simulink model "HybridPowertrain_TestBench_Final"  (R2017a)
settings: Solver=ode1  StartTime=0.0  StopTime=1400  FixedStep=0.01  RelTol=1e-3  EnableMultiTasking=on
undefined symbols (not defined in the file): AccActPos, air, Atm_temp, bms_inletair_temp, BMS_IstStrom, bms_maxchargecurrent, bms_maxdischargecurrent, BMS_Notfallkuehlung, BMS_SOC, BrkPdlPos, cal, Cells, Chg, D1_Commanded_Torque, D1_DC_Bus_Voltage, D2_Motor_Speed, D2_Torque_Feedback, DriverControls, EcoCAR3_Lib, Em, EngActStdyStTorq, Engine, EngSpd, env, ESS, fd, g, gb, Gearbox, GearBox, gps_lat, gps_long, Grade, I_loss, IMG, InstFuelConsmpRate, KeyPosition, lib_ESS_plant_V1_2, Loss, max_vehicle_rad_air_flow, mot, mph2kph, mph2ms, NeutralGear, ParkGear, PPEI_Engine_General_Status_2__ThrPos, PTEI_Engine_Torque_Status__EngActStdyStTorq, R_0, R_1, Ratio, RegenBrkDisable, rho, SampleTime, ShiftLeverPosition, SOC_bp, SOC_init, Spd, Speed, SW_CS_ON, SW_Engine_ON ... (+15)
libraries: simulink x39, fl_lib x13, nesl_utility x8, Utility x1, EC2_libraries x1
(part 3 of 5)

== system HybridPowertrain_TestBench_Final/ESS/Soft BMS/BMS_1 ==
  Bus Creator8 : BusCreator  Inputs=9
  Constant2 : Constant  Value=0
  BMS_06 : Outport
  wires:
  ? -> Bus Creator8/5
  ? -> Bus Creator8/9
  ? -> Bus Creator8/7
  ? -> Bus Creator8/3
  ? -> Bus Creator8/4
  ? -> Bus Creator8/6
  ? -> Bus Creator8/8
  Bus Creator8/1 -> BMS_06/1  "BMS_06"
  Constant2/1 -> Bus Creator8/2  "BMS_SollVolumenStrom"

== system HybridPowertrain_TestBench_Final/ESS/Soft BMS/BMS_2 ==
  Bus Creator8 : BusCreator  Inputs=9
  BMS_07 : Outport
  wires:
  ? -> Bus Creator8/2
  Bus Creator8/1 -> BMS_07/1  "BMS_07"
  ? -> Bus Creator8/8
  ? -> Bus Creator8/6
  ? -> Bus Creator8/4
  ? -> Bus Creator8/3
  [BMS_Gesamtst_Spgfreiheit] -> Bus Creator8/1  "BMS_Gesamtst_Spgfreiheit"
  ? -> Bus Creator8/7
  ? -> Bus Creator8/9
  ? -> Bus Creator8/5

== system HybridPowertrain_TestBench_Final/ESS/Soft BMS/BMS_3 ==
  Bus Creator8 : BusCreator  Inputs=3
  Constant : Constant  Value=255
  Constant1 : Constant  Value=254
  Data Type Conversion : DataTypeConversion
  ISO_Hybrid_01_Resp : Outport
  wires:
  Bus Creator8/1 -> ISO_Hybrid_01_Resp/1  "ISO_Hybrid_01_Resp"
  Data Type Conversion/1 -> Bus Creator8/1  "ISO_Hybrid_01_Resp_Data_4"
  Constant/1 -> Bus Creator8/2  "ISO_Hybrid_01_Resp_Data_5"
  Constant1/1 -> Bus Creator8/3  "ISO_Hybrid_01_Resp_Data_6"
  [ISO_Hybrid_01_Req_Data_4] -> Data Type Conversion/1  "ISO_Hybrid_01_Resp_Data_4"

== system HybridPowertrain_TestBench_Final/ESS/Soft BMS/BMS_HYB_1 ==
  BMS_HYB_02_BZ : Subsystem
  Bus Creator3 : BusCreator  Inputs=20
  Clock3 : Clock  Commented=on
  Constant12 : Constant  Value=0
  Constant7 : Constant  Value=0
  Constant8 : Constant  Value=0
  Data Type Conversion : DataTypeConversion
  Speed1 : Lookup  Commented=on  InputValues=[0 75 75 100 100 120]  Table=[0 0 1 1 0 0]
  BMS_HYB_02 : Outport
  wires:
  [BMS_SleepInd] -> Bus Creator3/17  "BMS_SleepInd"
  [BMS_Fehler_Notabschaltung_Pilot] -> Bus Creator3/16  "BMS_Fehler_Notabschaltung_Pilot"
  [BMS_Init_abgeschlossen] -> Bus Creator3/15  "BMS_Init_abgeschlossen"
  Constant12/1 -> Bus Creator3/14  "BMS_Fehler_Kaltstartleistung"
  [BMS_IstSpannung] -> Bus Creator3/13  "BMS_IstSpannung"
  [BMS_Fehler_verschweisst] -> Bus Creator3/12  "BMS_Fehler_HS_verschweisst"
  [BMS_Fehler_HS_offen] -> Bus Creator3/11  "BMS_Fehler_HS_offen"
  [BMS_IstStrom] -> Bus Creator3/10  "BMS_IstStrom"
  [BMS_Fehler_Pilot] -> Bus Creator3/9  "BMS_Fehler_Pilot"
  [BMS_Gesamtst_Spgfreiheit] -> Bus Creator3/4  "BMS_Status_Spgfreiheit"
  [BMS_Fehler_Notabschaltung_Crash] -> Bus Creator3/5  "BMS_Fehler_Notabschaltung_Crash"
  Constant8/1 -> Bus Creator3/8  "BMS_Fehler_Isolation"
  [BMS_Notfallkuehlung] -> Bus Creator3/2  "BMS_Notfallkuehlung"
  Constant7/1 -> Bus Creator3/7  "BMS_Fehler_HVBattAbschaltung_Anf"
  [BMS_Fehler_Notabschaltung_Crash] -> Bus Creator3/6  "BMS_Fehler_HVBattAbschaltung"
  [BMS_Gesamtst_Spgfreiheit] -> Bus Creator3/3  "BMS_Status_Spannungsfreiheit"
  Data Type Conversion/1 -> Bus Creator3/1  "BMS_IstModus"
  Bus Creator3/1 -> BMS_HYB_02/1  "BMS_HYB_02"
  Clock3/1 -> Speed1/1
  [BMS_IstModus] -> Data Type Conversion/1  "BMS_IstModus"
  BMS_HYB_02_BZ/1(Out1) -> Bus Creator3/18

== system HybridPowertrain_TestBench_Final/ESS/Soft BMS/BMS_HYB_2 ==
  Bus Creator3 : BusCreator  Inputs=10
  Data Type Conversion : DataTypeConversion
  BMS_HYB_03 : Outport
  wires:
  Bus Creator3/1 -> BMS_HYB_03/1  "BMS_HYB_03"
  Data Type Conversion/1 -> Bus Creator3/1  "BMS_SOC"
  [BMS_SOC] -> Data Type Conversion/1  "BMS_SOC"

== system HybridPowertrain_TestBench_Final/ESS/Soft BMS/BMS_HYB_3 ==
  Bus Creator6 : BusCreator  Inputs=9
  Constant : Constant
  Constant1 : Constant  Commented=on  Value=bms_maxdischargecurrent
  Constant2 : Constant
  Constant3 : Constant  Commented=on  Value=bms_maxchargecurrent
  BMS_HYB_04 : Outport
  wires:
  Constant2/1 -> Bus Creator6/2
  [BMS_Spannung_ZwKr] -> Bus Creator6/3  "BMS_Spannung_ZwKr"
  ? -> Bus Creator6/7
  ? -> Bus Creator6/9
  ? -> Bus Creator6/8
  ? -> Bus Creator6/5
  ? -> Bus Creator6/4
  ? -> Bus Creator6/6
  Bus Creator6/1 -> BMS_HYB_04/1  "BMS_HYB_04"
  Constant/1 -> Bus Creator6/1  "BMS_MaxDyn_LadeStrom"

== system HybridPowertrain_TestBench_Final/ESS/Soft BMS/BMS_HYB_4 ==
  Bus Creator6 : BusCreator  Inputs=9
  Constant1 : Constant  Value=430
  Constant2 : Constant  Value=291
  Constant3 : Constant  Value=0
  Constant4 : Constant  Commented=on  Value=bms_inletair_temp
  Constant5 : Constant  Value=20
  BMS_HYB_06 : Outport
  wires:
  Constant5/1 -> Bus Creator6/5  "BMS_Temperatur_Ansaugluft"
  [BMS_Temperatur] -> Bus Creator6/4  "BMS_Temperatur"
  Constant3/1 -> Bus Creator6/1  "BMS_Balancing_Anf"
  Bus Creator6/1 -> BMS_HYB_06/1  "BMS_HYB_06"
  ? -> Bus Creator6/6
  Constant2/1 -> Bus Creator6/3  "BMS_Min_EntladeSpannung"
  ? -> Bus Creator6/8
  ? -> Bus Creator6/9
  ? -> Bus Creator6/7
  Constant1/1 -> Bus Creator6/2  "BMS_Max_LadeSpannung"

== system HybridPowertrain_TestBench_Final/ESS/Soft BMS/BMS_HYB_5 ==
  Bus Creator6 : BusCreator  Inputs=9
  BMS_HYB_07 : Outport
  wires:
  ? -> Bus Creator6/7
  ? -> Bus Creator6/9
  ? -> Bus Creator6/8
  ? -> Bus Creator6/5
  ? -> Bus Creator6/4
  ? -> Bus Creator6/6
  Bus Creator6/1 -> BMS_HYB_07/1  "BMS_HYB_07"
  [BMS_Temperierung_Anf] -> Bus Creator6/1  "BMS_Temperierung_Anf"

== system HybridPowertrain_TestBench_Final/ESS/Soft BMS/BMS_Hybrid_1 ==
  Bus Creator8 : BusCreator  Inputs=1
  BMS_Hybrid_01 : Outport
  wires:
  [BMS_HYB_Kuehlung_Anf] -> Bus Creator8/1  "BMS_HYB_Kuehlung_Anf"
  Bus Creator8/1 -> BMS_Hybrid_01/1  "BMS_Hybrid_01"

== system HybridPowertrain_TestBench_Final/ESS/Soft BMS/Energy Consumption ==
  Current : Inport
  Voltage : Inport  Port=2
  Divide : Product  Inputs=*/
  Divide by zero : Subsystem
  Gain : Gain  Gain=mph2kph
  Initial Current1 : Memory  InheritSampleTime=on
  Multiply : Product  Inputs=**
  Sum5 : Sum  Inputs=|++  SaturateOnIntegerOverflow=on  InputSameDT=on  OutDataTypeStr=Inherit: Same as first input
  To Workspace4 : ToWorkspace  VariableName=ess_wh_per_km  SampleTime=-1
      settings: Decimation=WORKSPACE_DECIMATION
  To_WHr1 : Gain  Gain=tloop/3600  SaturateOnIntegerOverflow=on  OutDataTypeStr=Inherit: Same as input  ParamDataTypeStr=Inherit: Same as input
  tag scope: ESSPwr=global
  wires:
  Current/1 -> Multiply/1
  Voltage/1 -> Multiply/2
  Multiply/1 -> [ESSPwr], To_WHr1/1  "Power"
  To_WHr1/1 -> Sum5/1  "d(Wh)"
  Sum5/1 -> Initial Current1/1  "Wh"
  Initial Current1/1 -> Sum5/2, Divide/1  "Wh"
  [veh_dist_miles] -> Gain/1  "mi"
  Divide/1 -> To Workspace4/1  "Wh/km"
  Gain/1 -> Divide by zero/1(In1)  "km"
  Divide by zero/1(Out1) -> Divide/2

== system HybridPowertrain_TestBench_Final/ESS/Soft BMS/HV_Netz status ==
  ess_vbat : Inport
  Constant3 : Constant  Value=2
  Constant4 : Constant
  Constant5 : Constant  Value=0
  Constant6 : Constant  Value=0
  Memory : Memory
  Memory1 : Memory
  Switch : Switch  Criteria=u2 > Threshold  Threshold=20
  Switch1 : Switch  Threshold=1
  Switch2 : Switch  Threshold=7
  BMS_Spannung_Zwkr : Outport
  BMS_Gesamtst_Spgfreiheit : Outport  Port=2
  wires:
  Constant5/1 -> Switch1/3
  [BMS_IstModus] -> Switch1/2, Switch2/2
  Switch1/1 -> Memory/1
  Constant6/1 -> Switch2/1
  Switch2/1 -> Memory1/1
  Constant4/1 -> Switch/3
  Switch/1 -> BMS_Gesamtst_Spgfreiheit/1
  Constant3/1 -> Switch/1
  ess_vbat/1 -> Switch1/1
  Memory/1 -> Switch2/3
  Memory1/1 -> BMS_Spannung_Zwkr/1, Switch/2

== system HybridPowertrain_TestBench_Final/ESS/Soft BMS/Limits ==
  vcell : Inport
  Average Current : Subsystem
  Compare To Constant1 : simulink/Logic and Bit Operations/Compare To Constant  relop=<=  const=3.0  OutDataTypeStr=boolean
  Compare To Constant2 : simulink/Logic and Bit Operations/Compare To Constant  relop=<=  const=3.0  OutDataTypeStr=boolean
  Constant3 : Constant  Value=25
  Derate : Subsystem
  Derate2 : Subsystem
  Gain : Gain  Gain=1/1.9
  Gain1 : Gain  Gain=1/1.9
  To Workspace10 : ToWorkspace  VariableName=ess_dis_max_current_underated  SampleTime=-1
      settings: Decimation=WORKSPACE_DECIMATION
  To Workspace3 : ToWorkspace  VariableName=ess_dis_max  SampleTime=-1
      settings: Decimation=WORKSPACE_DECIMATION
  To Workspace4 : ToWorkspace  VariableName=ess_chg_max  SampleTime=-1
      settings: Decimation=WORKSPACE_DECIMATION
  To Workspace9 : ToWorkspace  VariableName=ess_chg_max_current_underated  SampleTime=-1
      settings: Decimation=WORKSPACE_DECIMATION
  bcm_chg_max_tbl : Lookup2D  RowIndex=ess.plant.init.limit.idx1_soc  ColumnIndex=ess.plant.init.limit.idx2_temp  Table=ess.plant.init.max_charge_limit
  bcm_dis_max_tbl : Lookup2D  RowIndex=ess.plant.init.limit.idx1_soc  ColumnIndex=ess.plant.init.limit.idx2_temp  Table=ess.plant.init.max_discharge_limit
  bcm_dis_max : Outport
  bcm_chg_max : Outport  Port=2
  Discharge Buffer : Outport  Port=3
  Charge Buffer : Outport  Port=4
  t_coolant : Outport  Port=5
  undervolt : Outport  Port=6
  overvolt : Outport  Port=7
  tag scope: bcm_chg_max=global
  wires:
  [BMS_Temperatur] -> bcm_chg_max_tbl/2, bcm_dis_max_tbl/2, Average Current/2(Temp)
  bcm_dis_max_tbl/1 -> Gain/1
  Derate/1(Derate) -> bcm_dis_max/1, To Workspace3/1
  bcm_chg_max_tbl/1 -> Gain1/1  "bcm_chg_max"
  Derate2/1(Derate) -> To Workspace4/1, [bcm_chg_max], bcm_chg_max/1
  [BMS_SOC] -> Average Current/1(SOC), bcm_dis_max_tbl/1, bcm_chg_max_tbl/1
  Average Current/1(Discharge Buffer) -> Derate/2(Buffer), Discharge Buffer/1
  Average Current/2(Discharge Cont) -> Derate/3(Cont Current)
  Average Current/3(Charge Buffer) -> Derate2/1(Buffer), Charge Buffer/1
  Average Current/4(Charge Cont) -> Derate2/2(Cont Current)
  vcell/1 -> Compare To Constant1/1, Compare To Constant2/1
  Constant3/1 -> t_coolant/1
  Compare To Constant2/1 -> overvolt/1
  Compare To Constant1/1 -> undervolt/1
  Gain/1 -> Derate/1(Current Limit), To Workspace10/1
  Gain1/1 -> To Workspace9/1, Derate2/3(Current Limit)

== system HybridPowertrain_TestBench_Final/ESS/Soft BMS/NMH_BMS1 ==
  Bus Creator8 : BusCreator  Inputs=9
  NMH_BMS : Outport
  wires:
  [NMH_BMS_Start_1] -> Bus Creator8/3  "NMH_BMS_Start_1"
  [NMH_BMS_Normal_Mode_2] -> Bus Creator8/2  "NMH_BMS_Normal_Mode_2"
  Bus Creator8/1 -> NMH_BMS/1  "NMH_BMS"
  ? -> Bus Creator8/8
  ? -> Bus Creator8/6
  [NMH_BMS_Start_2] -> Bus Creator8/4  "NMH_BMS_Start_2"
  [NMH_BMS_Normal_Mode_1] -> Bus Creator8/1  "NMH_BMS_Normal_Mode_1"
  ? -> Bus Creator8/7
  ? -> Bus Creator8/9
  [NMH_BMS_Car_WakeUp] -> Bus Creator8/5  "NMH_BMS_Car_WakeUp"

== system HybridPowertrain_TestBench_Final/ESS/Soft BMS/NoiseAdd ==
  In : Inport
  Random Number : RandomNumber  Variance=0.1  SampleTime=tloop
  Rate Transition : RateTransition
  Sum : Sum  Inputs=|++
  Out : Outport
  wires:
  Random Number/1 -> Rate Transition/1
  In/1 -> Sum/1
  Sum/1 -> Out/1
  Rate Transition/1 -> Sum/2

== system HybridPowertrain_TestBench_Final/ESS/Soft BMS/RollingAliveCnt1 ==
  Constant : Constant
  Rolling Alive Counter : Stateflow chart  TreatAsAtomicUnit=on
  Switch : Switch  Criteria=u2 > Threshold
  Out1 : Outport
  wires:
  Switch/1 -> Out1/1
  [BMS_CAN_fault] -> Switch/2
  Rolling Alive Counter/1(RollingAliveCnt) -> Switch/3
  Constant/1 -> Switch/1

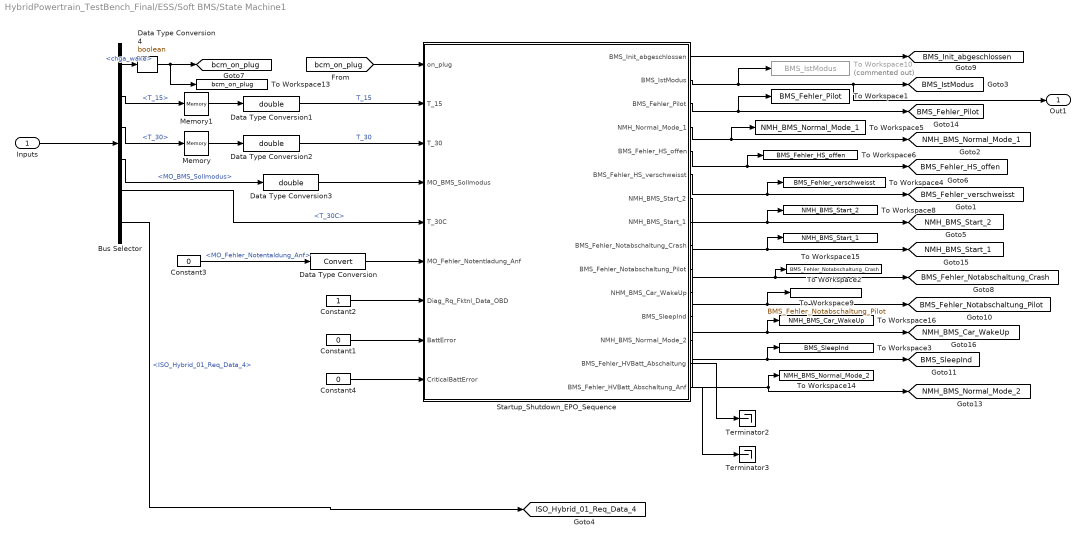
== system HybridPowertrain_TestBench_Final/ESS/Soft BMS/State Machine1 ==
  Inputs : Inport
  Bus Selector : BusSelector  OutputSignals=chga_wake,T_15,T_30,MO_BMS_Sollmodus,T_30C,ISO_Hybrid_01_Req_Data_4
  Constant1 : Constant  Value=0  OutDataTypeStr=boolean
  Constant2 : Constant  OutDataTypeStr=boolean
  Constant3 : Constant  Value=0  OutDataTypeStr=boolean
  Constant4 : Constant  Value=0  OutDataTypeStr=boolean
  Data Type Conversion : DataTypeConversion
  Data Type Conversion1 : DataTypeConversion  OutDataTypeStr=double
  Data Type Conversion2 : DataTypeConversion  OutDataTypeStr=double
  Data Type Conversion3 : DataTypeConversion  OutDataTypeStr=double
  Data Type Conversion4 : DataTypeConversion  OutDataTypeStr=boolean
  Memory : Memory  InheritSampleTime=on
  Memory1 : Memory  InheritSampleTime=on
  Startup_Shutdown_EPO_Sequence : Stateflow chart  TreatAsAtomicUnit=on
  Terminator2 : Terminator
  Terminator3 : Terminator
  To Workspace1 : ToWorkspace  VariableName=BMS_Fehler_Pilot  SampleTime=-1
      settings: Decimation=WORKSPACE_DECIMATION
  To Workspace10 : ToWorkspace  Commented=on  VariableName=BMS_IstModus  SampleTime=-1
      settings: Decimation=WORKSPACE_DECIMATION
  To Workspace13 : ToWorkspace  VariableName=bcm_on_plug  SampleTime=-1
      settings: Decimation=WORKSPACE_DECIMATION
  To Workspace14 : ToWorkspace  VariableName=NMH_BMS_Normal_Mode_2  SampleTime=-1
      settings: Decimation=WORKSPACE_DECIMATION
  To Workspace15 : ToWorkspace  VariableName=NMH_BMS_Start_1  SampleTime=-1
      settings: Decimation=WORKSPACE_DECIMATION
  To Workspace16 : ToWorkspace  VariableName=NMH_BMS_Car_WakeUp  SampleTime=-1
      settings: Decimation=WORKSPACE_DECIMATION
  To Workspace2 : ToWorkspace  VariableName=BMS_Fehler_Notabschaltung_Crash  SampleTime=-1
      settings: Decimation=WORKSPACE_DECIMATION
  To Workspace3 : ToWorkspace  VariableName=BMS_SleepInd  SampleTime=-1
      settings: Decimation=WORKSPACE_DECIMATION
  To Workspace4 : ToWorkspace  VariableName=BMS_Fehler_verschweisst  SampleTime=-1
      settings: Decimation=WORKSPACE_DECIMATION
  To Workspace5 : ToWorkspace  VariableName=NMH_BMS_Normal_Mode_1  SampleTime=-1
      settings: Decimation=WORKSPACE_DECIMATION
  To Workspace6 : ToWorkspace  VariableName=BMS_Fehler_HS_offen  SampleTime=-1
      settings: Decimation=WORKSPACE_DECIMATION
  To Workspace8 : ToWorkspace  VariableName=NMH_BMS_Start_2  SampleTime=-1
      settings: Decimation=WORKSPACE_DECIMATION
  To Workspace9 : ToWorkspace  VariableName=BMS_Fehler_Notabschaltung_Pilot  SampleTime=-1
      settings: Decimation=WORKSPACE_DECIMATION
  Out1 : Outport
  tag scope: BMS_Fehler_HS_offen=global, BMS_Fehler_Notabschaltung_Crash=global, BMS_Fehler_Notabschaltung_Pilot=global, BMS_Fehler_Pilot=global, BMS_Fehler_verschweisst=global, BMS_Init_abgeschlossen=global, BMS_IstModus=global, BMS_SleepInd=global, ISO_Hybrid_01_Req_Data_4=global, NMH_BMS_Car_WakeUp=global, NMH_BMS_Normal_Mode_1=global, NMH_BMS_Normal_Mode_2=global, NMH_BMS_Start_1=global, NMH_BMS_Start_2=global, bcm_on_plug=global
  wires:
  Data Type Conversion4/1 -> [bcm_on_plug], To Workspace13/1
  Data Type Conversion3/1 -> Startup_Shutdown_EPO_Sequence/4(MO_BMS_Sollmodus)
  Memory1/1 -> Data Type Conversion1/1
  Memory/1 -> Data Type Conversion2/1
  Data Type Conversion2/1 -> Startup_Shutdown_EPO_Sequence/3(T_30)  "T_30"
  Data Type Conversion1/1 -> Startup_Shutdown_EPO_Sequence/2(T_15)  "T_15"
  Data Type Conversion/1 -> Startup_Shutdown_EPO_Sequence/6(MO_Fehler_Notentladung_Anf)
  Bus Selector/4 -> Data Type Conversion3/1  "<MO_BMS_Sollmodus>"
  Inputs/1 -> Bus Selector/1
  Startup_Shutdown_EPO_Sequence/15(BMS_Fehler_HVBatt_Abschaltung_Anf) -> Terminator3/1
  Startup_Shutdown_EPO_Sequence/14(BMS_Fehler_HVBatt_Abschaltung) -> Terminator2/1
  Constant4/1 -> Startup_Shutdown_EPO_Sequence/9(CriticalBattError)
  Constant2/1 -> Startup_Shutdown_EPO_Sequence/7(Diag_Rq_Fktnl_Data_OBD)
  Constant1/1 -> Startup_Shutdown_EPO_Sequence/8(BattError)
  Constant3/1 -> Data Type Conversion/1  "<MO_Fehler_Notentaldung_Anf>"
  Bus Selector/5 -> Startup_Shutdown_EPO_Sequence/5(T_30C)  "<T_30C>"
  [bcm_on_plug] -> Startup_Shutdown_EPO_Sequence/1(on_plug)
  Startup_Shutdown_EPO_Sequence/11(NHM_BMS_Car_WakeUp) -> [NMH_BMS_Car_WakeUp], To Workspace16/1
  Startup_Shutdown_EPO_Sequence/8(NMH_BMS_Start_1) -> To Workspace15/1, [NMH_BMS_Start_1]
  Startup_Shutdown_EPO_Sequence/7(NMH_BMS_Start_2) -> [NMH_BMS_Start_2], To Workspace8/1
  Startup_Shutdown_EPO_Sequence/13(NMH_BMS_Normal_Mode_2) -> [NMH_BMS_Normal_Mode_2], To Workspace14/1
  Startup_Shutdown_EPO_Sequence/3(BMS_Fehler_Pilot) -> [BMS_Fehler_Pilot], To Workspace1/1
  Startup_Shutdown_EPO_Sequence/1(BMS_Init_abgeschlossen) -> [BMS_Init_abgeschlossen]
  Startup_Shutdown_EPO_Sequence/2(BMS_IstModus) -> To Workspace10/1, [BMS_IstModus], Out1/1
  Bus Selector/2 -> Memory1/1  "<T_15>"
  Startup_Shutdown_EPO_Sequence/6(BMS_Fehler_HS_verschweisst) -> To Workspace4/1, [BMS_Fehler_verschweisst]
  Startup_Shutdown_EPO_Sequence/4(NMH_Normal_Mode_1) -> [NMH_BMS_Normal_Mode_1], To Workspace5/1
  Startup_Shutdown_EPO_Sequence/9(BMS_Fehler_Notabschaltung_Crash) -> [BMS_Fehler_Notabschaltung_Crash], To Workspace2/1
  Startup_Shutdown_EPO_Sequence/10(BMS_Fehler_Notabschaltung_Pilot) -> [BMS_Fehler_Notabschaltung_Pilot], To Workspace9/1
  Startup_Shutdown_EPO_Sequence/5(BMS_Fehler_HS_offen) -> [BMS_Fehler_HS_offen], To Workspace6/1
  Startup_Shutdown_EPO_Sequence/12(BMS_SleepInd) -> [BMS_SleepInd], To Workspace3/1
  Bus Selector/1 -> Data Type Conversion4/1  "<chga_wake>"
  Bus Selector/3 -> Memory/1  "<T_30>"
  Bus Selector/6 -> [ISO_Hybrid_01_Req_Data_4]  "<ISO_Hybrid_01_Req_Data_4>"

== system HybridPowertrain_TestBench_Final/ESS/Soft BMS/Temperature Management ==
  ess_temp : Inport
  Add2 : Sum  Inputs=+-
  Constant : Constant
  Constant1 : Constant  Value=3
  Constant2 : Constant  Commented=on  Value=BMS_Notfallkuehlung
  Constant3 : Constant
  K : Constant  Value=273.15
  Switch : Switch
  tag scope: BMS_HYB_Kuehlung_Anf=global, BMS_Temperatur=global, BMS_Temperierung_Anf=global
  wires:
  Constant/1 -> Switch/1
  Switch/1 -> [BMS_HYB_Kuehlung_Anf], [BMS_Temperierung_Anf]
  Constant1/1 -> Switch/3
  Constant3/1 -> [BMS_Notfallkuehlung]
  ess_temp/1 -> Add2/1, Switch/2
  K/1 -> Add2/2
  Add2/1 -> [BMS_Temperatur]

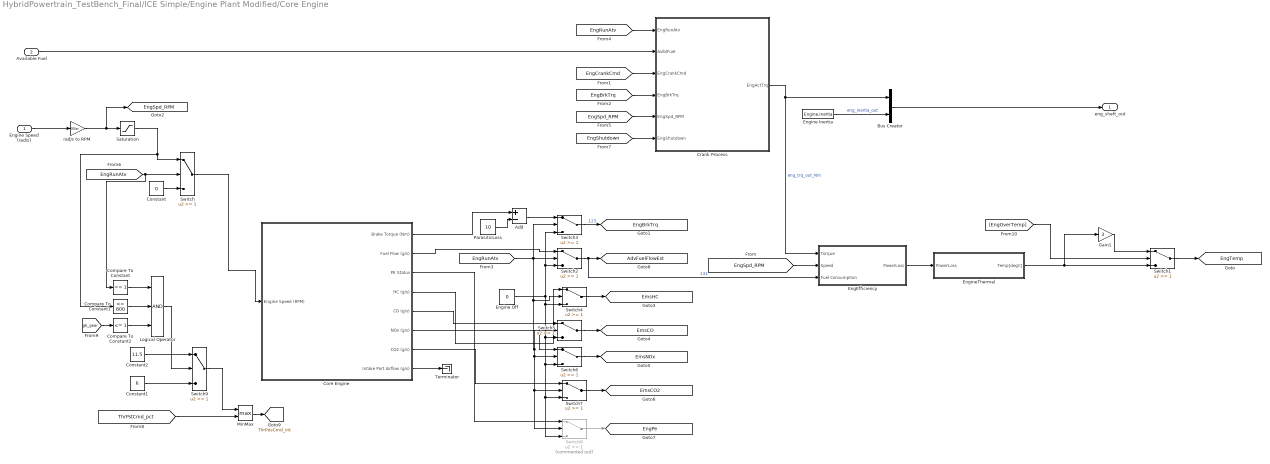
== system HybridPowertrain_TestBench_Final/ICE Simple/Engine Plant Modified/Core Engine ==
  Engine Speed (rad/s) : Inport
  Available Fuel : Inport  Port=2
  Add : Sum  Inputs=+-
  Bus Creator : BusCreator  Inputs=2
  Compare To Constant : simulink/Logic and Bit Operations/Compare To Constant  relop===  const=1  OutDataTypeStr=boolean
  Compare To Constant1 : simulink/Logic and Bit Operations/Compare To Constant  relop=<=  const=800  OutDataTypeStr=boolean
  Compare To Constant2 : simulink/Logic and Bit Operations/Compare To Constant  relop=<=  const=1  OutDataTypeStr=boolean
  Constant : Constant  Value=0
  Constant1 : Constant  Value=6
  Constant2 : Constant  Value=11.5
  Core Engine : Subsystem
      mask Display: image(imread('EngineShortBlock.jpg'),'center')
  Crank Process : Stateflow chart  TreatAsAtomicUnit=on
  EngEfficiency : Subsystem
  Engine Inertia : Constant  Value=Engine.Inertia
  "Engine Off  " : Constant  Value=0
  EngineThermal : Subsystem
  Gain1 : Gain  Gain=3
  Logical Operator : Logic  Inputs=3  AllPortsSameDT=off  OutDataTypeStr=boolean
  MinMax : MinMax  Function=max  Inputs=2
  ParasiticLoss : Constant  Value=10
  Saturation : Saturate  UpperLimit=max(Engine.Engine.TQ.SPEED)  LowerLimit=0
  Switch{,1..7,9} (9 alike) : Switch  Threshold=1
  Switch8 : Switch  Commented=on  Threshold=1
  Terminator : Terminator
  rad/s to RPM : Gain  Gain=30/pi
  eng_shaft_out : Outport
  tag scope: AdvFuelFlowEst=global, EmsCO2=global, EmsCO=global, EmsHC=global, EmsNOx=global, EngBrkTrq=global, EngPe=global, EngSpd_RPM=global, EngTemp=global, ThrPosCmd_int=global
  wires:
  [EngShutdown] -> Crank Process/6(EngShutdown)
  Saturation/1 -> Compare To Constant1/1, Switch/1
  [EngSpd_RPM] -> Crank Process/5(EngSpd_RPM)
  [EngCrankCmd] -> Crank Process/3(EngCrankCmd)
  [EngBrkTrq] -> Crank Process/4(EngBrkTrq)
  [EngRunAtv] -> Crank Process/1(EngRunAtv)
  Switch8/1 -> [EngPe]
  Switch7/1 -> [EmsCO2]
  Switch6/1 -> [EmsNOx]
  Switch5/1 -> [EmsCO]
  "Engine Off  "/1 -> Switch8/3, Switch7/3, Switch6/3, Switch5/3, Switch4/3, Switch2/3, Switch3/3
  [EngRunAtv] -> Switch8/2, Switch7/2, Switch6/2, Switch5/2, Switch4/2, Switch2/2, Switch3/2
  Switch4/1 -> [EmsHC]
  Switch3/1 -> [EngBrkTrq]  "123"
  Available Fuel/1 -> Crank Process/2(AvlblFuel)
  Switch2/1 -> EngEfficiency/3(Fuel Consumption), [AdvFuelFlowEst]  "131"
  Crank Process/1(EngActTrq) -> Bus Creator/1, EngEfficiency/1(Torque)  "eng_trq_out_Nm"
  Engine Inertia/1 -> Bus Creator/2  "eng_inertia_out"
  Bus Creator/1 -> eng_shaft_out/1
  [EngRunAtv] -> Switch/2, Compare To Constant/1
  Constant/1 -> Switch/3
  rad/s to RPM/1 -> [EngSpd_RPM], Saturation/1
  EngEfficiency/1(PowerLoss) -> EngineThermal/1(PowerLoss)
  EngineThermal/1(Temp[degC]) -> Gain1/1, Switch1/3
  Engine Speed (rad/s)/1 -> rad/s to RPM/1
  [EngSpd_RPM] -> EngEfficiency/2(Speed)
  [EngOverTemp] -> Switch1/2
  Gain1/1 -> Switch1/1
  Switch1/1 -> [EngTemp]
  Core Engine/2(Fuel Flow (g/s)) -> Switch2/1
  Core Engine/3(PE Status) -> Switch8/1
  Core Engine/4(HC (g/s)) -> Switch4/1
  Core Engine/5(CO (g/s)) -> Switch5/1
  Core Engine/6(NOx (g/s)) -> Switch6/1
  Core Engine/7(CO2 (g/s)) -> Switch7/1
  Core Engine/8(Intake Port Airflow (g/s)) -> Terminator/1
  Switch/1 -> Core Engine/1(Engine Speed (RPM))
  Core Engine/1(Brake Torque (Nm)) -> Add/1
  Constant2/1 -> Switch9/1
  Compare To Constant/1 -> Logical Operator/1
  Compare To Constant1/1 -> Logical Operator/2
  Logical Operator/1 -> Switch9/2
  [gb_gear] -> Compare To Constant2/1
  Compare To Constant2/1 -> Logical Operator/3
  [ThrPstCmd_pct] -> MinMax/2
  MinMax/1 -> [ThrPosCmd_int]
  Constant1/1 -> Switch9/3
  Switch9/1 -> MinMax/1
  ParasiticLoss/1 -> Add/2
  Add/1 -> Switch3/1

== system HybridPowertrain_TestBench_Final/ICE Simple/Engine Plant Modified/ECU Actuators ==
  In1 : Inport
  Bus Selector : BusSelector  OutputSignals=ThrPosCmd_%,Eng12vStrtrMtrCmmdOn,EngRunAtv,FuelPumpEnable,EngShutdown,Eng_Temp,fan_cmd,VehSpdAvgDrvn
  Out1 : Outport
  Out2 : Outport  Port=2
  Out3 : Outport  Port=3
  Out4 : Outport  Port=4
  Out5 : Outport  Port=5
  Out6 : Outport  Port=6
  Out7 : Outport  Port=7
  Out8 : Outport  Port=8
  wires:
  Bus Selector/5 -> Out5/1  "<EngShutdown>"
  Bus Selector/4 -> Out4/1  "<FuelPumpEnable>"
  In1/1 -> Bus Selector/1
  Bus Selector/1 -> Out1/1  "<ThrPosCmd_%>"
  Bus Selector/2 -> Out2/1  "<Eng12vStrtrMtrCmmdOn>"
  Bus Selector/3 -> Out3/1  "<EngRunAtv>"
  Bus Selector/6 -> Out6/1  "<Eng_Temp>"
  Bus Selector/7 -> Out7/1  "<fan_cmd>"
  Bus Selector/8 -> Out8/1  "<VehSpdAvgDrvn>"

== system HybridPowertrain_TestBench_Final/ICE Simple/Engine Plant Modified/ECU Sensors ==
  In1 : Inport
  In2 : Inport  Port=2
  In3 : Inport  Port=3
  In4 : Inport  Port=4
  In5 : Inport  Port=5
  In6 : Inport  Port=6
  In7 : Inport  Port=7
  In8 : Inport  Port=8
  In9 : Inport  Port=9
  In10 : Inport  Port=10
  Bus Creator : BusCreator  Inputs=10
  Memory : Memory
  Out1 : Outport
  wires:
  In9/1 -> Bus Creator/9  "NOx_g/s"
  In1/1 -> Bus Creator/1  "EngActStdyStTorq_Nm"
  In2/1 -> Bus Creator/2  "EngSpd_RPM"
  In3/1 -> Bus Creator/3  "EngFuelFlow_g/s"
  In4/1 -> Bus Creator/4  "FuelLevelPct"
  In5/1 -> Bus Creator/5  "PE_0_1"
  In6/1 -> Bus Creator/6  "HC_g/s"
  In7/1 -> Bus Creator/7  "CO_g/s"
  Bus Creator/1 -> Memory/1
  In8/1 -> Bus Creator/8  "CO2_g/s"
  In10/1 -> Bus Creator/10  "Eng_Temp"
  Memory/1 -> Out1/1

== system HybridPowertrain_TestBench_Final/ICE Simple/Engine Plant Modified/Fuel Supply ==
  0 to 100 : Saturate
  Fuel Pump Disable : Constant  Value=0
  Fuel Volumn : Constant  Value=Engine.Fuel.Initial_Volumn
  Integrator : Integrator  LimitOutput=on  UpperSaturationLimit=Engine.FuelTank.Volume  LowerSaturationLimit=0
  L to % : Gain  Gain=100/Engine.FuelTank.Volume
  Sum : Sum  Inputs=+-
  Switch : Switch  Threshold=1
  g to L : Gain  Gain=1/Engine.Fuel.Density/1000
  Available Fuel : Outport
  tag scope: FuelLevelPct=global
  wires:
  0 to 100/1 -> [FuelLevelPct]
  L to %/1 -> 0 to 100/1
  Fuel Pump Disable/1 -> Switch/3
  g to L/1 -> Switch/1
  Integrator/1 -> g to L/1
  [AdvFuelFlowEst] -> Integrator/1
  [FuelPumpEnable] -> Switch/2
  Sum/1 -> Available Fuel/1, L to %/1
  Switch/1 -> Sum/2
  Fuel Volumn/1 -> Sum/1

== system HybridPowertrain_TestBench_Final/ICE Simple/Engine Plant Modified/Radiator ==
  note: Calculation of max air flow:
      |
      | The air flow reach the max in the scenario that only fan rejects all the heat coolant brings in
      |
      | The regular max CFM of a vehicle radiator fan is about 2000
      |
      | CFM=1.76* Q/delta T_air
      |
      | Where Q is the max amount of heat from coolant, assume that the max temperature drop of coolant
      | through radiator is 10 deg C
      |
      | Q= Mc_coolant* Cp_coolant* delta T_coolant=3500*0.26*10=9100w
      |
      | delta T_air=1.76*Q/CFM=1.76*9100/2000=8 degC
      |
      | Max Mc_air=Q/(Cp_air*delta T_air)=9100/(1006*8)=1.13 kg/s
  EngCltTmp : Inport
  Fans : Inport  Port=2
  " " : Product  Inputs=**
  " " : Gain  Gain=0.05
  Ambient Temp : Constant  Value=env.init.T_ambiant
  Compare To Zero : simulink/Logic and Bit Operations/Compare To Zero  relop=<=  OutDataTypeStr=boolean
  Constant : Constant
  Cp of Air : Constant  Value=air.init.specific_heat
  Cp of Air1 : Constant  Value=air.init.specific_heat
  Data Type Conversion1 : DataTypeConversion
  Divide by Zero Fix : Subsystem
  "Eng Mc=Q/(Cp*delta T) " : Product  Inputs=*/
  Q=Mc_air*Cp_air*delta T : Product  Inputs=***
  Saturation : Saturate  UpperLimit=max_vehicle_rad_air_flow  LowerLimit=-1
  Sum3 : Sum  Inputs=|-+
  Sum4 : Sum
  Sum5 : Sum  Inputs=|+-
  Switch : Switch  Threshold=1
  vehspdflow : Gain  Gain=0.01
  tag scope: AirFlowRequest=global, Heat_Reject_Eng=global
  wires:
  Data Type Conversion1/1 -> " "/1
  Cp of Air1/1 -> Q=Mc_air*Cp_air*delta T/3
  Switch/1 -> Q=Mc_air*Cp_air*delta T/2  "eng act air flow in kg/s"
  Q=Mc_air*Cp_air*delta T/1 -> " "/2  "J/s"
  " "/1 -> [Heat_Reject_Eng]  "J"
  Saturation/1 -> Sum3/1  "Actual air flow"
  Sum3/1 -> Compare To Zero/1
  Compare To Zero/1 -> Switch/2  "request meet"
  Cp of Air/1 -> "Eng Mc=Q/(Cp*delta T) "/2  "Cp J/kg*C"
  Ambient Temp/1 -> Sum5/2  "25 deg C"
  Sum5/1 -> Divide by Zero Fix/2(Divide), Q=Mc_air*Cp_air*delta T/1  "Delta T = Tcoolant - Tambient"
  EngCltTmp/1 -> Sum5/1  "EngCltTmp in deg C"
  "Eng Mc=Q/(Cp*delta T) "/1 -> Switch/1, Sum3/2, [AirFlowRequest]  "Eng requested air flow in Kg/s"
  Sum4/1 -> Switch/3, Saturation/1  "Air Flow Recieved"
  Fans/1 -> Data Type Conversion1/1
  [VehSpdAvgDrvn_Eng] -> vehspdflow/1
  vehspdflow/1 -> Sum4/2
  [Heat_Transfer_Eng] -> Divide by Zero Fix/1(Multiply)  "heat generation in w"
  Divide by Zero Fix/1(Output) -> "Eng Mc=Q/(Cp*delta T) "/1
  " "/1 -> Sum4/1
  Constant/1 -> " "/1

== system HybridPowertrain_TestBench_Final/ICE Simple/Inputs/Analog ==
  Out1 : Outport
  wires:
  [Analog] -> Out1/1

== system HybridPowertrain_TestBench_Final/ICE Simple/Inputs/CAN_from_HCU ==
  Bus Creator : BusCreator  Inputs=2
  Out1 : Outport
  wires:
  [HCU_to_EBCAN] -> Bus Creator/1
  [HCU_to_VEH_CAN] -> Bus Creator/2
  Bus Creator/1 -> Out1/1

== system HybridPowertrain_TestBench_Final/ICE Simple/Soft ECM/ECM_RollingAliveCnt ==
  Constant : Constant
  Rolling Alive Counter : Stateflow chart  TreatAsAtomicUnit=on
  Switch : Switch  Criteria=u2 > Threshold
  Out1 : Outport
  wires:
  [ECM_CAN_fault] -> Switch/2
  Constant/1 -> Switch/1
  Rolling Alive Counter/1(RollingAliveCnt) -> Switch/3
  Switch/1 -> Out1/1  "ECM_RollingAliveCnt"

== system HybridPowertrain_TestBench_Final/ICE Simple/Soft ECM/Fuel Consumption ==
  note: Total Fuel Consumed
  Fuel Consumption : Inport
  " " : Constant  Value=3600
  " tloop" : Constant  Value=0.01
  1/fuel density : Gain  Gain=1/(Engine.Fuel.Density*1000)
  Add : Sum  Inputs=|++
  Add1 : Sum  Inputs=|++
  Constant3 : Constant  Value=Engine.Fuel.Lower_Heating_Value/1000
  Divide : Product  Inputs=*/
  Divide by Zero Fix : Subsystem
  Divide by Zero Fix1 : Subsystem
  Memory : Memory
  Memory1 : Memory
  Product : Product  RndMeth=Zero
  Product1 : Product  RndMeth=Zero
  Product3 : Product  RndMeth=Zero
  Scope : Scope
  To Workspace5 : ToWorkspace  Commented=on  VariableName=eng_wh_per_mile_hist  SampleTime=-1
      settings: Decimation=WORKSPACE_DECIMATION
  fuel consumption : Outport
  wires:
  Divide by Zero Fix1/1(Output) -> To Workspace5/1
  Divide/1 -> Add1/1  "Wh"
  Memory1/1 -> Add1/2
  Add1/1 -> Divide by Zero Fix1/2(Multiply), Memory1/1  "cumulative"
  Product/1 -> Product3/2  "W"
  Constant3/1 -> Product/2
  Divide by Zero Fix/1(Output) -> fuel consumption/1, Scope/1
  [veh_dist_miles] -> Divide by Zero Fix1/1(Divide), Divide by Zero Fix/2(Multiply)  "miles"
  Product1/1 -> Add/1  "liter"
  1/fuel density/1 -> Product1/1  "liter/sec"
  Fuel Consumption/1 -> Product/1, 1/fuel density/1  "g/s"
  Memory/1 -> Add/2
  Add/1 -> Divide by Zero Fix/1(Divide), Memory/1  "cumulative_liter"
  " tloop"/1 -> Product3/1, Product1/2
  Product3/1 -> Divide/1
  " "/1 -> Divide/2

== system HybridPowertrain_TestBench_Final/ICE Simple/Soft ECM/Logic/APP2TP ==
  EngSpd : Inport
  APP : Inport  Port=2
  Shifter : Inport  Port=3
  f : TriggerPort  TriggerType=function-call  VariantControl=Variant
      settings: CopyFcn=Stateflow.SLINSF.SimulinkMan.removeBlockPreDeleteFcn  PreDeleteFcn=Stateflow.SLINSF.SimulinkMan.unsafePredeleteFcn
  Based on APP to TP test data from 2013 Malibu : Lookup_n-D  NumberOfTableDimensions=1  BreakpointsForDimension1=[0,1,2,3,4,5,6,7,8,9,10,11,12,13,14,15,16,17,18,19,20,21,22,23,24,25,26,27,28,29,30,31,32,33,34,35,36,37,38,39,40,41,42,43,44,45,46,48,51,55,60,66,100]  Table=[0,6.3,12.7686537241448,12.6326703204763,12.8888951657611,13.4307541011932,14.1739282202018,15.0532596030224,16.0198646102832,17.0384547356068,18.0848650172271,19.1437900086214,20.206727308158,21.2701286477589,22.3337585405773,23.3992604876916,24.4689307438132,25.5446996420107,26.6273204774486,27.7157659501418,28.8068321667249,29.8949502012373,30.9722052149229,32.0285631350456,33.0523048927199,34.0306682197568,34.9506970045247,35.8002982068255,36.5695063317874,37.2519554627699,37.846558853288,38.359396077948,38.8058077424007,39.2126977523099,39.6210431413345,40.0886114581279,40.6928857123509,41.5341968797017,42.7390639659588,44.4637416300428,46.8979753660875,50.2689642445339,54.8455312122302,60.9425009515619,68.9252852985734,79.2146762201353,81.9427,84.6943,87.2166,89.5096,91.3439,92.6051,100]  ExtrapMethod=Clip  UseLastTableValue=on  InternalRulePriority=Speed  RndMeth=Simplest  InputSameDT=on
  Compare To Constant : simulink/Logic and Bit Operations/Compare To Constant  relop=<=  const=Engine.IdleSpeed  OutDataTypeStr=boolean
  Compare To Constant1 : simulink/Logic and Bit Operations/Compare To Constant  relop=<=  const=3.0  OutDataTypeStr=boolean
  Constant : Constant  Value=ParkGear
  Constant1 : Constant  Value=NeutralGear
  Constant2 : Constant  Value=Engine.IdleSpeed
  Display : Display
  Divide : Product  Inputs=**
  "EngSpd " : InportShadow
  Kp : Gain  Gain=0.5
  Logical Operator : Logic  Operator=OR  Inputs=3  AllPortsSameDT=off  OutDataTypeStr=boolean
  Logical Operator1 : Logic  AllPortsSameDT=off  OutDataTypeStr=boolean
  Memory : Memory  InheritSampleTime=on
  Product : Product
  RPM Derating : Lookup_n-D  NumberOfTableDimensions=1  BreakpointsForDimension1=[0 1000 2000 3000 4000 5000 6000 7000]  Table=[1 1 1 1 1 1 1 0]  ExtrapMethod=Clip  UseLastTableValue=on  InternalRulePriority=Speed  RndMeth=Simplest  InputSameDT=on
  Relational Operator : RelationalOperator  Operator===  OutDataTypeStr=boolean  RndMeth=Nearest
  Relational Operator1 : RelationalOperator  Operator===  OutDataTypeStr=boolean  RndMeth=Nearest
  Sum : Sum  Inputs=|+-
  Switch : Switch  Threshold=1
  TP : Outport
  wires:
  Based on APP to TP test data from 2013 Malibu/1 -> Product/1  "1"
  EngSpd/1 -> Compare To Constant/1, RPM Derating/1
  RPM Derating/1 -> Product/2  "2"
  Shifter/1 -> Relational Operator/2, Relational Operator1/1
  Constant/1 -> Relational Operator/1
  Constant1/1 -> Relational Operator1/2
  Relational Operator/1 -> Logical Operator/1
  Relational Operator1/1 -> Logical Operator/2
  Logical Operator/1 -> Logical Operator1/1
  Constant2/1 -> Sum/1
  "EngSpd "/1 -> Sum/2
  Sum/1 -> Divide/2
  Divide/1 -> Memory/1, Switch/1
  Logical Operator1/1 -> ?  "Idle"
  Compare To Constant1/1 -> Logical Operator1/2
  APP/1 -> Display/1, Compare To Constant1/1, Based on APP to TP test data from 2013 Malibu/1  "3"
  Product/1 -> Switch/3
  Compare To Constant/1 -> Logical Operator/3
  Switch/1 -> TP/1
  Memory/1 -> Kp/1
  Kp/1 -> Divide/1

== system HybridPowertrain_TestBench_Final/IMG/IMG Plant/ Actuators ==
  In1 : Inport
  Bus Selector : BusSelector  OutputSignals=MotTrqCmd,Direction_Command,InverterEnabled
  Out2 : Outport
  Out3 : Outport  Port=2
  Out4 : Outport  Port=3
  wires:
  Bus Selector/1 -> Out2/1  "<MotTrqCmd>"
  In1/1 -> Bus Selector/1
  Bus Selector/2 -> Out3/1  "<Direction_Command>"
  Bus Selector/3 -> Out4/1  "<InverterEnabled>"

== system HybridPowertrain_TestBench_Final/IMG/IMG Plant/Calculate Mot Efficiency, MotPwrMech, and, MotPwrElec ==
  note: Pelec_req = Pmech_req*Eff^k,
      | k = -1 if Trq >= 0,
      | k = 1 if Trq < 0
  MotSpd : Inport
  MotTrqAct : Inport  Port=2
  -1 : Gain  Gain=8
  "-1 when + 1 when - " : Gain  Gain=-1
  -2 : Gain  Gain=tloop
  2-D Lookup Table : Lookup_n-D  BreakpointsForDimension1=mot.plant.init.eff_trq.idx2_trq  BreakpointsForDimension2=mot.plant.init.eff_trq.idx1_spd  Table=mot.plant.init.eff_trq.map  InternalRulePriority=Speed  RndMeth=Simplest  InputSameDT=on
  Abs{,1..3} (4 alike) : Abs
  Add : Sum  Inputs=-+
  Add1 : Sum  Inputs=+-
  Add2 : Sum  Commented=on
  Constant : Constant  Value=1-mot.plant.init.mcu_eff
  Constant1 : Constant  Commented=on  Value=mot.plant.init.mcu_mass
  Constant2 : Constant  Commented=on  Value=mot.plant.init.specific_heat
  Divide : Product  Commented=on  Inputs=*/
  Gain2 : Gain  Gain=1/100
  Lower Limit : Subsystem  Commented=on  mask{Lolimit=t_amb+20}
      mask prompts: Lolimit "Lower Limit"
  MCUOverTemp Fault : Subsystem  Commented=on
  MCU_WEGPmp : Constant  Value=0
  Math Function1 : Math  Operator=pow  SaturateOnIntegerOverflow=on
  Memory : Memory
  Memory1 : Memory  Commented=on
  Product : Product
  Product1 : Product
  Product2 : Product
  Product3 : Product  Commented=on
  Sign : Signum
  rad/s to rpm : Gain  Gain=30/pi
  Losses : Outport
  MotPwrElec : Outport  Port=2
  MCU_Heat : Outport  Port=3
  wires:
  rad/s to rpm/1 -> Abs1/1
  Abs1/1 -> 2-D Lookup Table/2
  Sign/1 -> "-1 when + 1 when - "/1
  Abs/1 -> 2-D Lookup Table/1
  Gain2/1 -> Math Function1/1
  2-D Lookup Table/1 -> Gain2/1
  Product1/1 -> Product2/1, Add/2, MotPwrElec/1  "MotPwrElec"
  Product/1 -> Add/1, Product1/1  "MotPwrMech"
  MotTrqAct/1 -> Memory/1, Product/1, Abs/1
  MotSpd/1 -> Product/2, rad/s to rpm/1
  "-1 when + 1 when - "/1 -> Math Function1/2
  Abs2/1 -> Losses/1
  Add/1 -> Abs2/1
  Math Function1/1 -> Product1/2
  Memory/1 -> Sign/1
  Constant/1 -> Product2/2
  Product2/1 -> Abs3/1
  Abs3/1 -> Add1/1
  MCU_WEGPmp/1 -> -1/1
  Add1/1 -> -2/1
  -1/1 -> Add1/2
  -2/1 -> MCU_Heat/1
  Constant1/1 -> Product3/1
  Constant2/1 -> Product3/2
  Product3/1 -> Divide/2
  Divide/1 -> Add2/1
  Memory1/1 -> Add2/2
  Add2/1 -> Lower Limit/1(In1)
  Lower Limit/1(Out1) -> MCUOverTemp Fault/1(In1), Memory1/1

== system HybridPowertrain_TestBench_Final/IMG/IMG Plant/MotTrqExcessTrigger ==
  In1 : Inport
  Bias : Bias  Bias=55
  Bias1 : Bias  Bias=25
  Constant : Constant  Value=0
  Multiport Switch : MultiPortSwitch  DataPortOrder=Zero-based contiguous
  Out1 : Outport
  tag scope: MotTrqExcessTrig=global
  wires:
  Multiport Switch/1 -> Out1/1
  Bias/1 -> Multiport Switch/4
  In1/1 -> Multiport Switch/2, Bias/1, Bias1/1
  Bias1/1 -> Multiport Switch/3
  Constant/1 -> [MotTrqExcessTrig], Multiport Switch/1

== system HybridPowertrain_TestBench_Final/IMG/IMG Plant/Motor_Plant ==
  Trq_cmd : Inport
  Batt_volt : Inport  Port=2
  Speed_rad/sec : Inport  Port=3
  Add : Sum
  Bus Creator : BusCreator  Inputs=5
  Efficiency Calcs : Subsystem
  Memory : Memory
  Random Number : RandomNumber  Mean=0.1  Variance=0.1  SampleTime=0.01
  rad/sec to rpm : Gain  Gain=60/(2*3.14)
  Mot_out : Outport
  wires:
  Add/1 -> Memory/1
  Speed_rad/sec/1 -> rad/sec to rpm/1
  rad/sec to rpm/1 -> Bus Creator/2, Efficiency Calcs/1(Speed_rpm)  "Mot_spd_rpm"
  Random Number/1 -> Add/2
  Memory/1 -> Bus Creator/1, Efficiency Calcs/2(Torq_cmd_Nm)  "Mot_Trq_Nm"
  Bus Creator/1 -> Mot_out/1
  Trq_cmd/1 -> Add/1
  Batt_volt/1 -> Efficiency Calcs/3(Batt_volt)
  Efficiency Calcs/1(Mot_current) -> Bus Creator/3
  Efficiency Calcs/2(Mech_power_W) -> Bus Creator/4
  Efficiency Calcs/3(Elec_power_W) -> Bus Creator/5

== system HybridPowertrain_TestBench_Final/IMG/IMG Plant/Sensors ==
  In2 : Inport
  In3 : Inport  Port=2
  In4 : Inport  Port=3
  In5 : Inport  Port=4
  In6 : Inport  Port=5
  In1 : Inport  Port=6
  In7 : Inport  Port=7
  Bus Creator : BusCreator  Inputs=7
  Out1 : Outport
  wires:
  In6/1 -> Bus Creator/5  "mot_temp"
  In3/1 -> Bus Creator/2  "mot_trq_out"
  In5/1 -> Bus Creator/4  "mot_volt_in"
  In4/1 -> Bus Creator/3  "mot_crr_out"
  In2/1 -> Bus Creator/1  "mot_spd_out"
  Bus Creator/1 -> Out1/1
  In1/1 -> Bus Creator/6  "mcu_temp"
  In7/1 -> Bus Creator/7  "clt_plant_spd_in"

== system HybridPowertrain_TestBench_Final/IMG/IMG Plant/Thermal ==
  Losses : Inport
  Motor Thermal : Subsystem
  mot_temp_C : Outport
  wires:
  Losses/1 -> Motor Thermal/1(In1)  "[W]"
  Motor Thermal/1(Out1) -> mot_temp_C/1

== system HybridPowertrain_TestBench_Final/IMG/IMG Plant/Thermal1 ==
  Losses : Inport
  MCU_heat : Inport  Port=2
  MotInv_loop : Subsystem
  Motor Thermal : Subsystem  Commented=on
  MCU_temp_C : Outport
  motor_temp : Outport  Port=2
  wires:
  MCU_heat/1 -> MotInv_loop/2(In2)
  Losses/1 -> MotInv_loop/1(In1)  "[W]"
  MotInv_loop/1(Out1) -> MCU_temp_C/1
  MotInv_loop/2(Out2) -> motor_temp/1

== system HybridPowertrain_TestBench_Final/IMG/IMG Plant/Torque Calculation ==
  MotSpd : Inport
  MotTrqCmd : Inport  Port=2
  Abs : Abs
  Abs1 : Abs
  MinMax : MinMax  Inputs=2
  Product : Product
  Sign : Signum
  electric machine filter : Subsystem
  "max torque " : Subsystem
  mot_trq_out : Outport
  wires:
  "max torque "/1(max torque) -> Abs1/1
  MotSpd/1 -> "max torque "/2(speed)
  Sign/1 -> Product/1
  MinMax/1 -> Product/2
  Abs/1 -> MinMax/1
  Abs1/1 -> MinMax/2
  electric machine filter/1(filtered) -> mot_trq_out/1
  MotTrqCmd/1 -> "max torque "/1(cmd), Sign/1, Abs/1
  Product/1 -> electric machine filter/1(trq)

== system HybridPowertrain_TestBench_Final/IMG/IMG Plant/non-zero division ==
  note: original idea from Phil Sharer - ANL
      | original formula: u[1]\(u[2]+eps)*(u[2]!=0)
      | changes done by Gerald ZINI (dgey) - ANL (05\02\2001)
  note: (u[2]==0) is true then returns 1, thus (u[2]+(u[2]==0)) is equal to 0+1=1
  note: if u[2] == 0, then output == 0:
  note: (u[2]!=0) is false then returns 0
  note: and finally, the expression is: (u[1] \ 1) * 0 = 0
  note: (u[2]==0) is false then returns 0, thus (u[2]+(u[2]==0)) is equal to u[2]+0=u[2]
  note: if u[2] != 0, then output == u[1]\u[2]:
  note: (u[2]!=0) is true then returns 1
  note: and finally, the expression is: (u[1] \ u[2]) * 1 = u[1] \ u[2]
  In1 : Inport
  In2 : Inport  Port=2
  Fcn : Fcn  Expr=u[1]/(u[2]+(u[2]==0))*(u[2]!=0)
  Mux : Mux  Inputs=2
  Out1 : Outport
  wires:
  Mux/1 -> Fcn/1
  In1/1 -> Mux/1
  Fcn/1 -> Out1/1
  In2/1 -> Mux/2

== system HybridPowertrain_TestBench_Final/IMG/Soft MCU/MCU_CAN_rolling ==
  Constant8 : Constant
  Rolling Alive Counter1 : Stateflow chart  TreatAsAtomicUnit=on
  Switch1 : Switch  Criteria=u2 > Threshold
  Out1 : Outport
  wires:
  Switch1/1 -> Out1/1  "MCURollingAliveCnt [0 1 2 3]"
  [MCU_CAN_fault] -> Switch1/2
  Constant8/1 -> Switch1/1
  Rolling Alive Counter1/1(RollingAliveCnt) -> Switch1/3

== system HybridPowertrain_TestBench_Final/IMG/Soft MCU/Torque Calculation ==
  MotTrqReq : Inport
  MotSpd : Inport  Port=2
  MotTrqFdbck : Inport  Port=3
  Abs : Abs
  Abs1 : Abs
  MinMax : MinMax  Inputs=2
  Product : Product
  Sign : Signum
  "max torque " : Subsystem
  mot_trq_out : Outport
  wires:
  Product/1 -> mot_trq_out/1
  "max torque "/1(max torque) -> Abs1/1
  MotSpd/1 -> "max torque "/2(speed)
  MotTrqReq/1 -> "max torque "/1(Req), Sign/1, Abs/1
  Sign/1 -> Product/1
  MinMax/1 -> Product/2
  Abs/1 -> MinMax/1
  Abs1/1 -> MinMax/2
  MotTrqFdbck/1 -> "max torque "/3(torque)

== system HybridPowertrain_TestBench_Final/Measurements_stock/DriverControls/Clamping circuit ==
  preSat : Inport  DisableCoverage=on  SampleTime=SampleTime
  preIntegrator : Inport  DisableCoverage=on  Port=2  SampleTime=SampleTime
  AND : Logic  DisableCoverage=on  SampleTime=SampleTime
  DataTypeConv1 : DataTypeConversion  DisableCoverage=on  OutDataTypeStr=int8  SaturateOnIntegerOverflow=on  RndMeth=Zero  LockScale=on
  DataTypeConv2 : DataTypeConversion  DisableCoverage=on  OutDataTypeStr=int8  SampleTime=SampleTime
  DeadZone : DeadZone  DisableCoverage=on  LowerValue=LowerSaturationLimit  UpperValue=UpperSaturationLimit  SampleTime=SampleTime
  Equal : RelationalOperator  DisableCoverage=on  Operator===  SampleTime=SampleTime  RndMeth=Nearest  InputSameDT=on
  Memory : Memory  DisableCoverage=on
  NotEqual : RelationalOperator  DisableCoverage=on  Operator=~=  SampleTime=SampleTime  RndMeth=Nearest  InputSameDT=on
  SignDeltaU : Signum  DisableCoverage=on
  SignPreIntegrator : Signum  DisableCoverage=on  SampleTime=SampleTime
  ZeroGain : Gain  DisableCoverage=on  Gain=0  SaturateOnIntegerOverflow=on  OutDataTypeStr=Inherit: Same as input  ParamDataTypeStr=Inherit: Same as input
  Clamp : Outport  DisableCoverage=on  SampleTime=SampleTime
  wires:
  preSat/1 -> ZeroGain/1, DeadZone/1
  preIntegrator/1 -> SignPreIntegrator/1
  ZeroGain/1 -> NotEqual/1
  DeadZone/1 -> NotEqual/2, SignDeltaU/1
  SignDeltaU/1 -> DataTypeConv1/1
  DataTypeConv1/1 -> Equal/1
  SignPreIntegrator/1 -> DataTypeConv2/1
  DataTypeConv2/1 -> Equal/2
  NotEqual/1 -> AND/1
  Equal/1 -> AND/2
  AND/1 -> Memory/1
  Memory/1 -> Clamp/1

== system HybridPowertrain_TestBench_Final/Transmission/Inputs/Analog_fromHCU ==
  Outputs : Outport
  wires:
  [Analog] -> Outputs/1

== system HybridPowertrain_TestBench_Final/Transmission/Inputs/CAN_fromHCU ==
  Outputs : Outport
  wires:
  [HCU_to_VEH_CAN] -> Outputs/1

== system HybridPowertrain_TestBench_Final/Transmission/Inputs/Digital_fromHCU ==
  Outputs : Outport
  wires:
  [Digital] -> Outputs/1

== system HybridPowertrain_TestBench_Final/Transmission/Soft TCM/6L45 Logic/Gearbox_Control.Shift_Schedule.PlotShiftSchedule ==
  f : TriggerPort  TriggerType=function-call  VariantControl=Variant
      settings: CopyFcn=Stateflow.SLINSF.SimulinkMan.removeBlockPreDeleteFcn  PreDeleteFcn=Stateflow.SLINSF.SimulinkMan.unsafePredeleteFcn
  Subsystem : Subsystem
      settings: OpenFcn=|
      | figure;
      | PlotGearShiftSchedule(Gearbox.L45.PedalPositions,Gearbox.L45.UpShiftSpeeds,Gearbox.L45.DownShiftSpeeds,'6L45')
      mask Display: disp('Plot')

== system HybridPowertrain_TestBench_Final/Transmission/Soft TCM/6L45 Logic/Gearbox_Control.Shift_Schedule.calc_down ==
  Gear : Inport
  APP : Inport  Port=2
  f : TriggerPort  TriggerType=function-call  VariantControl=Variant
      settings: CopyFcn=Stateflow.SLINSF.SimulinkMan.removeBlockPreDeleteFcn  PreDeleteFcn=Stateflow.SLINSF.SimulinkMan.unsafePredeleteFcn
  Calculate Downshift Threshold : Lookup2D  RowIndex=gb.ctrl.dmd.init.gear_dnshift.idx1_lin_accel  ColumnIndex=[2,3,4,5,6,7,8]  Table=gb.ctrl.dmd.init.gear_dnshift.map'  LookUpMeth=Interpolation-Use End Values
  down_th : Outport
  wires:
  APP/1 -> Calculate Downshift Threshold/1
  Gear/1 -> Calculate Downshift Threshold/2
  Calculate Downshift Threshold/1 -> down_th/1

== system HybridPowertrain_TestBench_Final/Transmission/Soft TCM/6L45 Logic/Gearbox_Control.Shift_Schedule.calc_up ==
  Gear : Inport
  APP : Inport  Port=2
  f : TriggerPort  TriggerType=function-call  VariantControl=Variant
      settings: CopyFcn=Stateflow.SLINSF.SimulinkMan.removeBlockPreDeleteFcn  PreDeleteFcn=Stateflow.SLINSF.SimulinkMan.unsafePredeleteFcn
  Calculate Upshift Threshold : Lookup2D  RowIndex=gb.ctrl.dmd.init.gear_upshift.idx1_lin_accel  ColumnIndex=[1,2,3,4,5,6,7]  Table=gb.ctrl.dmd.init.gear_upshift.map'  LookUpMeth=Interpolation-Use End Values
  up_th : Outport
  wires:
  Gear/1 -> Calculate Upshift Threshold/2
  APP/1 -> Calculate Upshift Threshold/1
  Calculate Upshift Threshold/1 -> up_th/1

== system HybridPowertrain_TestBench_Final/Transmission/Soft TCM/6L45 Logic/Torque_Converter_Control.calc_lockup ==
  Gear : Inport
  APP : Inport  Port=2
  f : TriggerPort  TriggerType=function-call  VariantControl=Variant
      settings: CopyFcn=Stateflow.SLINSF.SimulinkMan.removeBlockPreDeleteFcn  PreDeleteFcn=Stateflow.SLINSF.SimulinkMan.unsafePredeleteFcn
  Calculate Lockup Threshold : Lookup2D  RowIndex=cpl.ctrl.init.trqconv_lockup.idx1_lin_accel  ColumnIndex=cpl.ctrl.init.trqconv_lockup.idx2_gear  Table=cpl.ctrl.init.trqconv_lockup.map  LookUpMeth=Interpolation-Use End Values
  lockup_th : Outport
  wires:
  Gear/1 -> Calculate Lockup Threshold/2
  APP/1 -> Calculate Lockup Threshold/1
  Calculate Lockup Threshold/1 -> lockup_th/1

== system HybridPowertrain_TestBench_Final/Transmission/Soft TCM/6L45 Logic/Torque_Converter_Control.calc_unlock ==
  Gear : Inport
  APP : Inport  Port=2
  f : TriggerPort  TriggerType=function-call  VariantControl=Variant
      settings: CopyFcn=Stateflow.SLINSF.SimulinkMan.removeBlockPreDeleteFcn  PreDeleteFcn=Stateflow.SLINSF.SimulinkMan.unsafePredeleteFcn
  Calculate Unlock Threshold : Lookup2D  RowIndex=cpl.ctrl.init.trqconv_unlock.idx1_lin_accel  ColumnIndex=cpl.ctrl.init.trqconv_unlock.idx2_gear  Table=cpl.ctrl.init.trqconv_unlock.map  LookUpMeth=Interpolation-Use End Values
  unlock_th : Outport
  wires:
  Gear/1 -> Calculate Unlock Threshold/2
  APP/1 -> Calculate Unlock Threshold/1
  Calculate Unlock Threshold/1 -> unlock_th/1

== system HybridPowertrain_TestBench_Final/Transmission/Transmission Plant/ Actuators ==
  In1 : Inport
  Bus Selector : BusSelector  OutputSignals=TransEstGear,LockupCmd
  Out2 : Outport
  Out5 : Outport  Port=2
  wires:
  Bus Selector/2 -> Out5/1  "<LockupCmd>"
  Bus Selector/1 -> Out2/1  "<TransEstGear>"
  In1/1 -> Bus Selector/1

== system HybridPowertrain_TestBench_Final/Transmission/Transmission Plant/Gearbox ==
  TransEstGear : Inport
  gb_trq_in gb_inertia_in : Inport  Port=2
  gb_spd_out : Inport  Port=3
  Bus Creator : BusCreator  Inputs=2
  Bus Selector : BusSelector  OutputSignals=tc_trq_out,tc_inertia_out
  Engine Inertia : Constant  Value=Engine.Inertia
  Gear : Lookup  InputValues=gb.plant.init.gear.idx1_shifter  Table=gb.plant.init.gear.idx2_gear  LookUpMeth=Interpolation-Use End Values  OutDataTypeStr=double  SaturateOnIntegerOverflow=on
  Inertia Calculation : Subsystem
  Memory : Memory
  Speed Calculation : Subsystem
  Subsystem : Subsystem
  Subsystem1 : Subsystem  Commented=on
  Torque calculation : Subsystem
  gear ratio table : Lookup  InputValues=gb.plant.init.ratio.idx1_gear  Table=gb.plant.init.ratio.map  LookUpMeth=Interpolation-Use End Values  SaturateOnIntegerOverflow=on
  gb_trq_out gb_inertia_out : Outport
  gb_spd_in : Outport  Port=2
  tag scope: gb_gear=global, gb_inertia_in=global, gb_inertia_out=global, gb_spd_in=global, gb_spd_out=global, gb_trq_in=global, gb_trq_out=global, gb_trq_ratio=global
  wires:
  TransEstGear/1 -> Memory/1
  Bus Selector/1 -> [gb_trq_in], Speed Calculation/3(torque input), Torque calculation/3(" input torque")  "<tc_trq_out>"
  Gear/1 -> Speed Calculation/1(gear number), [gb_gear], gear ratio table/1, Inertia Calculation/2(gear number), Torque calculation/2(gear number)
  gb_spd_out/1 -> Torque calculation/1(speed out), [gb_spd_out], Speed Calculation/2(spd out)
  gb_trq_in gb_inertia_in/1 -> Bus Selector/1
  Speed Calculation/1(Speed) -> [gb_spd_in], gb_spd_in/1
  Inertia Calculation/1(Inertia) -> [gb_inertia_out], Bus Creator/2  "gb_inertia_out"
  Bus Creator/1 -> gb_trq_out gb_inertia_out/1
  gear ratio table/1 -> [gb_trq_ratio]
  Memory/1 -> Gear/1
  Torque calculation/1(torque_out) -> Subsystem/2(In2), Subsystem/1(In1)  "gb_trq_out"
  Subsystem/1(Out1) -> Bus Creator/1, [gb_trq_out]  "gb_trq_out"
  Engine Inertia/1 -> [gb_inertia_in]
  Bus Selector/2 -> Speed Calculation/4(Inertia Input), Inertia Calculation/1(Inertia_in)  "<tc_inertia_out>"

== system HybridPowertrain_TestBench_Final/Transmission/Transmission Plant/Sensors ==
  In2 : Inport
  In3 : Inport  Port=2
  In4 : Inport  Port=3
  In5 : Inport  Port=4
  In6 : Inport  Port=5
  In7 : Inport  Port=6
  In1 : Inport  Port=7
  Bus Creator : BusCreator  Inputs=7
  Out1 : Outport
  wires:
  In7/1 -> Bus Creator/6  "TrnsOutShftTrq"
  In6/1 -> Bus Creator/5  "TrnsOutShftAngVel"
  In3/1 -> Bus Creator/2  "turbine_spd_rads"
  In5/1 -> Bus Creator/4  "tc_trq_out"
  In4/1 -> Bus Creator/3  "tc_trq_in"
  In2/1 -> Bus Creator/1  "impeller_spd_rads"
  Bus Creator/1 -> Out1/1
  In1/1 -> Bus Creator/7  "gb_trq_ratio"
